simulink model "PSKDPSKSimulation"  (R2023a)
settings: Solver=VariableStepAuto  StartTime=0.0  StopTime=0.1  FixedStep=1/(5*9600)  RelTol=1e-3
libraries: commsink2 x4, dspfdesign x4, commutil2 x2, commchan3 x2, commrandsrc3 x1
settings Model: Creator=29399  LastModifiedBy=DeathWind
settings SolverCC: AlgebraicLoopSolver=TrustRegion
settings DebuggingCC: UnconnectedInputMsg=warning  UnconnectedOutputMsg=warning  UnconnectedLineMsg=warning
settings ModelReferenceCC: EnableRefExpFcnMdlSchedulingChecks=on
settings SFSimCC: CustomCodeUndefinedFunction=UseInterfaceOnly

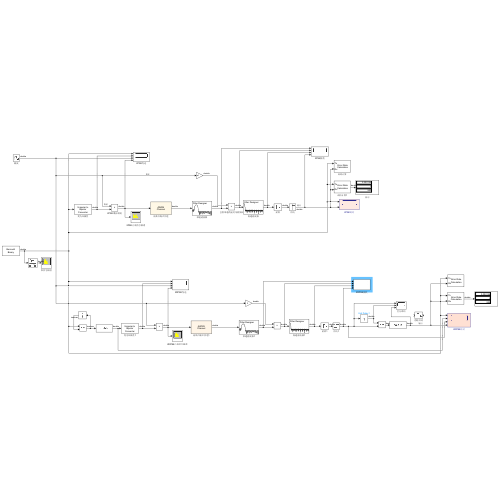
[thumbnail: Simulink's stored preview of the top-level diagram]
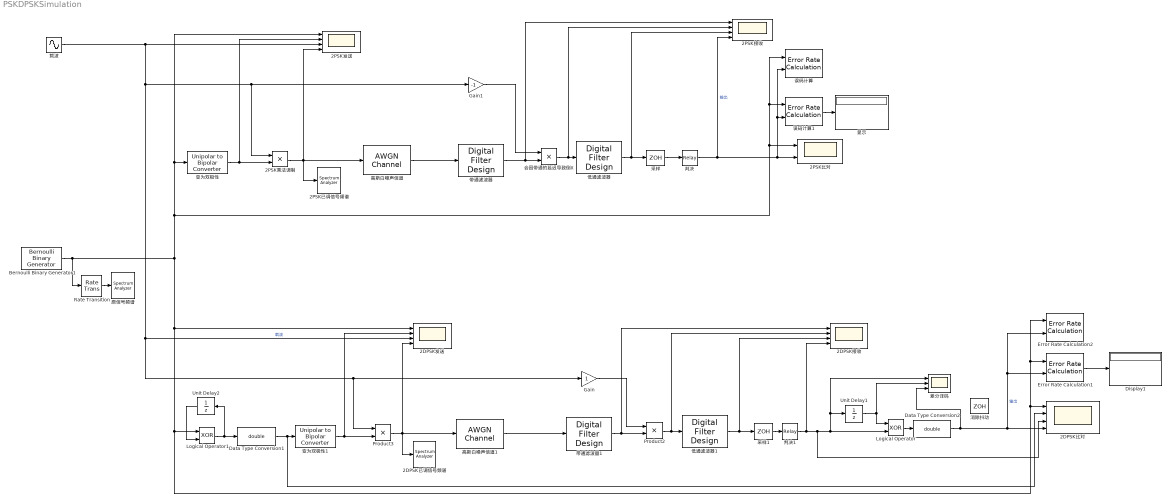
== system PSKDPSKSimulation ==
  2DPSK发送 : Scope  NumInputPorts=4
  2DPSK已调信号频谱 : SpectrumAnalyzer  WindowPosition=[184.000000,142.000000,1282.000000,700.000000,]  Visible=on  ScopeFrameLocation=window  Method=Welch  SampleRate=480000  PlotAsTwoSidedSpectrum=off  StartFrequency=0  StopFrequency=300e3  AveragingMethod=Running  SpectrumUnits=dBW  YLimits=[-101.13349971,-6.98841534]  DefaultConfigurationName=spbscopes.SpectrumAnalyzerBlockCfg  IsFrequencyInputMode=0  FrequencyVectorPort=0  FrequencyVectorFromPort=0  FrequencyInputRBWPort=0  FrequencyInputRBWFromPort=0
      settings: OpenAtSimulationStart=off
  2DPSK接收 : Scope  NumInputPorts=4
  2DPSK比对 : Scope  NumInputPorts=4
  2PSK乘法调制 : Product
  "2PSK发送 " : Scope  NumInputPorts=4
  "2PSK已调信号频谱 " : SpectrumAnalyzer  WindowPosition=[292.000000,139.000000,1282.000000,700.000000,]  Visible=on  ScopeFrameLocation=window  Method=Welch  SampleRate=480000  PlotAsTwoSidedSpectrum=off  StartFrequency=0  StopFrequency=300e3  AveragingMethod=Running  SpectrumUnits=dBW  Title=已调2PSK信号功率谱(未加噪)  YLimits=[-111.16841481,-2.86174807]  DefaultConfigurationName=spbscopes.SpectrumAnalyzerBlockCfg  IsFrequencyInputMode=0  FrequencyVectorPort=0  FrequencyVectorFromPort=0  FrequencyInputRBWPort=0  FrequencyInputRBWFromPort=0
      settings: OpenAtSimulationStart=off
  "2PSK接收 " : Scope  NumInputPorts=4
  2PSK比对 : Scope  NumInputPorts=2
  Bernoulli Binary Generator1 : commrandsrc3/Bernoulli Binary Generator  ProbabilityOfZero=0.5  SeedSource=Auto  Seed=0  SampleTime=1/9600  SamplesPerFrame=1  OutputDataType=double  SimulateUsing=Interpreted execution
  Data Type Conversion1 : DataTypeConversion  OutDataTypeStr=double  SaturateOnIntegerOverflow=off  RndMeth=Floor
  Data Type Conversion2 : DataTypeConversion  OutDataTypeStr=double  SaturateOnIntegerOverflow=off  RndMeth=Floor
  Display1 : Display
  Error Rate Calculation1 : commsink2/Error Rate Calculation  N=2  st_delay=0  cp_mode=Entire frame  subframe=[]  PMode=Port  WsName=ErrorVec  RsMode2=off  stop=off  numErr=100  maxBits=1e6
  Error Rate Calculation2 : commsink2/Error Rate Calculation  N=2  st_delay=0  cp_mode=Entire frame  subframe=[]  PMode=Workspace  WsName=Error2DPSK  RsMode2=off  stop=off  numErr=100  maxBits=1e6
  Gain : Gain
  Gain1 : Gain  Gain=-1
  Logical Operator : Logic  Operator=XOR  AllPortsSameDT=off  OutDataTypeStr=boolean
  Logical Operator1 : Logic  Operator=XOR  AllPortsSameDT=off  OutDataTypeStr=boolean
  Product2 : Product
  Product3 : Product
  Rate Transition : RateTransition  OutPortSampleTime=1/(5*9600)
  Unit Delay1 : UnitDelay  SampleTime=1/9600  HasFrameUpgradeWarning=on
  Unit Delay2 : UnitDelay  SampleTime=1/9600  HasFrameUpgradeWarning=on
  会因带通的延迟导致倒π : Product
  低通滤波器 : dspfdesign/Digital Filter Design  mwdsp_browser_bugfix_var=off
  低通滤波器1 : dspfdesign/Digital Filter Design  mwdsp_browser_bugfix_var=off
  "判决 " : Relay  OnSwitchValue=0  OffSwitchValue=0  OutMin=-1  OutMax=1
  判决1 : Relay  OnSwitchValue=0  OffSwitchValue=0
  "原信号频谱 " : SpectrumAnalyzer  WindowPosition=[408.000000,86.000000,1282.000000,700.000000,]  Visible=on  ScopeFrameLocation=window  Method=Welch  SampleRate=48000  PlotAsTwoSidedSpectrum=off  StartFrequency=20  StopFrequency=100e3  AveragingMethod=Running  YLimits=[-86.33757104,36.80114749]  DefaultConfigurationName=spbscopes.SpectrumAnalyzerBlockCfg  IsFrequencyInputMode=0  FrequencyVectorPort=0  FrequencyVectorFromPort=0  FrequencyInputRBWPort=0  FrequencyInputRBWFromPort=0
      settings: OpenAtSimulationStart=off
  变为双极性 : commutil2/Unipolar to Bipolar Converter  M=2  polarity=Positive  dataType=Inherit via internal rule
  变为双极性1 : commutil2/Unipolar to Bipolar Converter  M=2  polarity=Positive  dataType=Inherit via internal rule
  差分译码 : Scope  NumInputPorts=3
  带通滤波器 : dspfdesign/Digital Filter Design  mwdsp_browser_bugfix_var=off
  带通滤波器1 : dspfdesign/Digital Filter Design  mwdsp_browser_bugfix_var=off
  "显示 " : Display
  消除抖动 : ZeroOrderHold  SampleTime=1/9600
  误码计算 : commsink2/Error Rate Calculation  N=2  st_delay=0  cp_mode=Entire frame  subframe=[]  PMode=Workspace  WsName=Error2PSK  RsMode2=off  stop=off  numErr=100  maxBits=1e6
  误码计算1 : commsink2/Error Rate Calculation  N=2  st_delay=0  cp_mode=Entire frame  subframe=[]  PMode=Port  WsName=ErrorVec  RsMode2=off  stop=off  numErr=100  maxBits=1e6
  载波 : Sin  Frequency=5*9600*2*pi  SampleTime=1/(10*5*9600)
  采样 : ZeroOrderHold  SampleTime=1/9600
  采样1 : ZeroOrderHold  SampleTime=1/9600
  高斯白噪声信道 : commchan3/AWGN Channel  LegacyMode=on  NoiseMethod="Signal to noise ratio  (SNR)"  noiseMode="Signal to noise ratio  (SNR)"  EbNo=EbNo  EsNo=10  SNR=1  BitsPerSymbol=1  SignalPower=1  SamplesPerSymbol=1  SymbolPeriod=1/(5*9600)  VarianceSource=Parameter  Variance=1  RandomStream=Global stream  Seed=1234  SimulateUsing=Code generation
  高斯白噪声信道1 : commchan3/AWGN Channel  LegacyMode=on  NoiseMethod="Signal to noise ratio  (SNR)"  noiseMode="Signal to noise ratio  (SNR)"  EbNo=EbNo  EsNo=10  SNR=1  BitsPerSymbol=1  SignalPower=1  SamplesPerSymbol=1  SymbolPeriod=1/(5*9600)  VarianceSource=Parameter  Variance=1  RandomStream=Global stream  Seed=1234  SimulateUsing=Code generation
  wires:
  变为双极性/1 -> 2PSK乘法调制/2, "2PSK发送 "/2
  载波/1 -> "2PSK发送 "/3, Gain1/1, 2PSK乘法调制/1, 2DPSK发送/3, Gain/1, Product3/1  "载波"
  会因带通的延迟导致倒π/1 -> "2PSK接收 "/2, 低通滤波器/1
  2PSK乘法调制/1 -> 高斯白噪声信道/1, "2PSK已调信号频谱 "/1, "2PSK发送 "/4
  变为双极性1/1 -> Product3/2, 2DPSK发送/2
  Product2/1 -> 2DPSK接收/2, 低通滤波器1/1
  Product3/1 -> 高斯白噪声信道1/1, 2DPSK发送/4, 2DPSK已调信号频谱/1
  Data Type Conversion1/1 -> 2DPSK比对/2, 变为双极性1/1
  Logical Operator1/1 -> Data Type Conversion1/1, Unit Delay2/1
  Logical Operator/1 -> Data Type Conversion2/1
  Unit Delay1/1 -> Logical Operator/1, 差分译码/2
  Unit Delay2/1 -> Logical Operator1/2
  高斯白噪声信道1/1 -> 带通滤波器1/1
  带通滤波器1/1 -> 2DPSK接收/1, Product2/2
  带通滤波器/1 -> "2PSK接收 "/1, 会因带通的延迟导致倒π/2
  低通滤波器/1 -> 采样/1, "2PSK接收 "/3
  高斯白噪声信道/1 -> 带通滤波器/1
  Error Rate Calculation1/1 -> Display1/1
  误码计算1/1 -> "显示 "/1
  判决1/1 -> Unit Delay1/1, 差分译码/1, Logical Operator/2, 2DPSK比对/3, 2DPSK接收/4
  低通滤波器1/1 -> 采样1/1, 2DPSK接收/3
  Data Type Conversion2/1 -> 2DPSK比对/4, Error Rate Calculation1/2, Error Rate Calculation2/2, 差分译码/3  "输出"
  采样1/1 -> 判决1/1
  采样/1 -> "判决 "/1
  "判决 "/1 -> 误码计算/2, 误码计算1/2, 2PSK比对/2, "2PSK接收 "/4  "输出"
  Gain1/1 -> 会因带通的延迟导致倒π/1
  Gain/1 -> Product2/1
  Bernoulli Binary Generator1/1 -> Rate Transition/1, "2PSK发送 "/1, 变为双极性/1, 误码计算/1, 误码计算1/1, 2PSK比对/1, Error Rate Calculation2/1, Error Rate Calculation1/1, 2DPSK比对/1, Logical Operator1/1, 2DPSK发送/1
  Rate Transition/1 -> "原信号频谱 "/1
